simulink model "Simscape_crane_software_model"  (R2016b)
settings: Solver=ode15s  StartTime=0.0  StopTime=3  RelTol=1e-3  EnableMultiTasking=on
values from neighbouring files (symbols this model uses):
  m = 0.47    [SSmodelParams.mat]
  MR = 1.71    [SSmodelParams.mat]
  TxBreak = 0    [setup.m]
  TxCoulomb = 2.5    [setup.m]
  TxVisc = 49.1750    (= 49.175)    [setup.m]
  TyBreak = 0    [setup.m]
  TyCoulomb = 1.8    [setup.m]
  xZero = 0    [setup.m]
  yZero = 0    [setup.m]
undefined symbols (not defined in the file or in its folder): sigbuilder_block, TzBreak, TzCoulomb, X, xRange, Y, yRange, Z, zRange, zZero
undefined symbols (not defined in the file): M, TorqueMultX, TorqueMultY, TorqueMultZ, TxTrans, TyTrans, TyVisc, TzTrans, TzVisc
libraries: sm_lib x146, fl_lib x62, nesl_utility x24, elec_lib x9, simulink x6, sm_double_wishbone_suspension_lib x4, aerolibtransform2 x1
(part 1 of 14)
settings Model: Creator=jsustare  LastModifiedBy=Omar
settings SolverCC: MaxConsecutiveMinStep=10
settings DataIOCC: SaveFormat=StructureWithTime
settings OptimizationCC: LifeSpan=inf
settings DebuggingCC: AllowSymbolicDim=off  SFUnexpectedBacktrackingDiag=warning  SFNoUnconditionalDefaultTransitionDiag=warning  SFExecutionAtInitializationDiag=none
settings ModelReferenceCC: PropagateSignalLabelsOutOfModel=off
settings GRTTargetCC: TargetLangStandard=C89/C90 (ANSI)
settings ConfigComp: CovMetricSettings=dw  CovHtmlReporting=on  CovSaveCumulativeToWorkspaceVar=on  CovSaveSingleToWorkspaceVar=on  CovExternalEMLEnable=off
settings SimscapeCC: SimscapeLogType=all
settings ConfigurationSet: Description=SimMechanics 2G

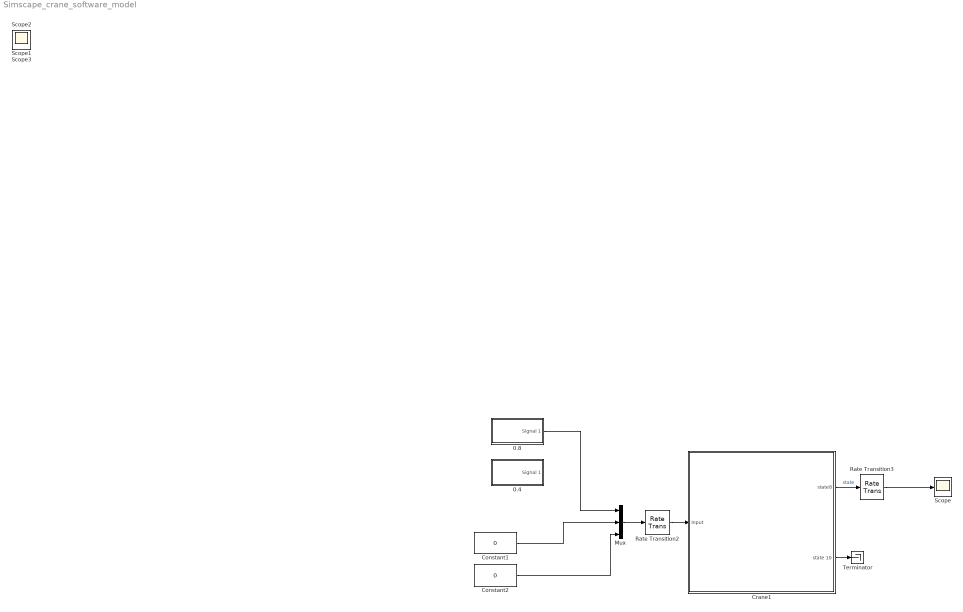
== system Simscape_crane_software_model ==
  0.4 : Subsystem  Tag=STV Subsys  LoadFcn=sigbuilder_block('load');  StartFcn=sigbuilder_block('start');  StopFcn=sigbuilder_block('stop');  ClipboardFcn=sigbuilder_block('clipboard');  mask(Sigbuilder block){tuvar=[0:10]}
      mask help: Simulink:masks:SigbuilderBlock_MD
      mask init:
      | if ~strcmp(get_param(bdroot(gcbh),'SimulationStatus'),'stopped') tuvar = sigbuilder_block('maskInit'); end
      settings: CopyFcn=sigbuilder_block('copy');  DeleteFcn=sigbuilder_block('delete');  ModelCloseFcn=sigbuilder_block('modelClose');  PreSaveFcn=sigbuilder_block('preSave');  PauseFcn=sigbuilder_block('pause');  ContinueFcn=sigbuilder_block('continue');  NameChangeFcn=sigbuilder_block('namechange');  OpenFcn=sigbuilder_block('open',[437.6 199.2 550.4 400 ]);  CloseFcn=sigbuilder_block('close');
      mask Display: plot(0, 0, 100, 100,[2, 2, 32, 32, 2], [68, 8, 8, 68, 68],[32, 2], [38, 38], [32, 19, 2],[53, 60, 44], [32, 17, 17, 2],[16, 16, 31, 31]);txt = getActiveGroup(gcbh);text(2, 100, txt,'verticalAlignment', 'top');
  0.8 : Subsystem  Tag=STV Subsys  LoadFcn=sigbuilder_block('load');  StartFcn=sigbuilder_block('start');  StopFcn=sigbuilder_block('stop');  ClipboardFcn=sigbuilder_block('clipboard');  mask(Sigbuilder block){tuvar=[0:10]}
      mask help: Simulink:masks:SigbuilderBlock_MD
      mask init:
      | if ~strcmp(get_param(bdroot(gcbh),'SimulationStatus'),'stopped') tuvar = sigbuilder_block('maskInit'); end
      settings: CopyFcn=sigbuilder_block('copy');  DeleteFcn=sigbuilder_block('delete');  ModelCloseFcn=sigbuilder_block('modelClose');  PreSaveFcn=sigbuilder_block('preSave');  PauseFcn=sigbuilder_block('pause');  ContinueFcn=sigbuilder_block('continue');  NameChangeFcn=sigbuilder_block('namechange');  OpenFcn=sigbuilder_block('open',[437.6 199.2 550.4 400 ]);  CloseFcn=sigbuilder_block('close');
      mask Display: plot(0, 0, 100, 100,[2, 2, 32, 32, 2], [68, 8, 8, 68, 68],[32, 2], [38, 38], [32, 19, 2],[53, 60, 44], [32, 17, 17, 2],[16, 16, 31, 31]);txt = getActiveGroup(gcbh);text(2, 100, txt,'verticalAlignment', 'top');
  Constant1 : Constant  Value=0
  Constant2 : Constant  Value=0
  Crane1 : Subsystem  mask{penduMass=m, cartMass=M, MR=MR, xRange=xRange, yRange=yRange, zRange=zRange, xZero=xZero, yZero=yZero, zZero=zZero, TxBreak=TxBreak, TxCoulomb=TxCoulomb, TxVisc=TxVisc, TxTrans=TxTrans, TyBreak=TyBreak, TyCoulomb=TyCoulomb, TyVisc=TyVisc, TyTrans=TyTrans, TzBreak=TzBreak, TzCoulomb=TzCoulomb, TzVisc=TzVisc, TzTrans=TzTrans, Ux=TorqueMultX, Uy=TorqueMultY, Uz=TorqueMultZ}
      mask prompts: penduMass "Pendulum Mass (Kg)"; cartMass "Mass of the cart (Kg)"; MR "Mass of the rail (Kg)"; TxBreak "BreakAwayFriction"; TxCoulomb "Coulomb Friction"; TxVisc "Viscous friction"; TxTrans "Transition coeff"; TyBreak "BreakAwayFriction"; TyCoulomb "Coulomb Friction"; TyVisc "Viscous friction"; TyTrans "Transition coeff"; TzBreak "BreakAwayFriction"; TzCoulomb "Coulomb Friction"; TzVisc "Viscous friction"; TzTrans "Transition coeff"; Ux "Rail motor multiplier (X)"; Uy "Cart motor multiplier (Y)"; Uz "String motor multiplier (Z)"
      mask init:
      | %mass lowSat
      | penduMass=max(penduMass,1e-3);
      | cartMass=max(cartMass,1e-3);
      | MR=max(MR,1e-3);
      | 
      | %zeros saturated
      | xZero=max(xZero,xRange(1));
      | xZero=min(xZero,xRange(2));
      | 
      | yZero=max(yZero,yRange(1));
      | yZero=min(yZero,yRange(2));
      | 
      | zZero=max(zZero,zRange(1));
      | zZero=min(zZero,zRange(2));
      mask DialogControl DescGroupVar Prompt: 3D Crane Simscape model
      mask Display:
